simulink model "Controlador2"  (R2026a)
settings: Solver=VariableStepAuto  StopTime=tfin
values from neighbouring files (symbols this model uses):
  tesc = 5    [CodigoTurner.m]    (also in CodigoTurnerPerturbacion.m; FiguraModeloH.m; FiguraModeloMoro.m; FiguraModeloTurner.m)
libraries: slpidlib x1, realtime_pacer_lib x1
settings Model: Creator=Nehir RT  LastModifiedBy=Nehir RT

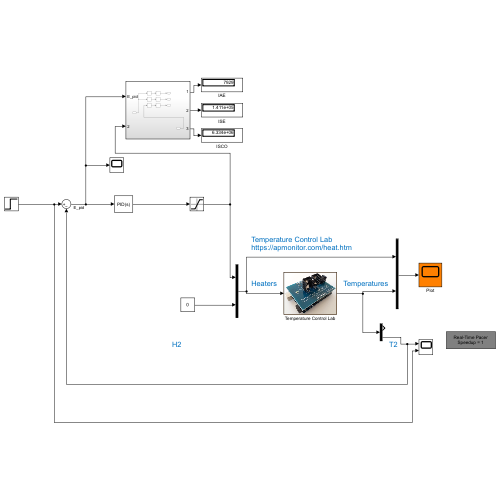
[thumbnail: Simulink's stored preview of the top-level diagram]
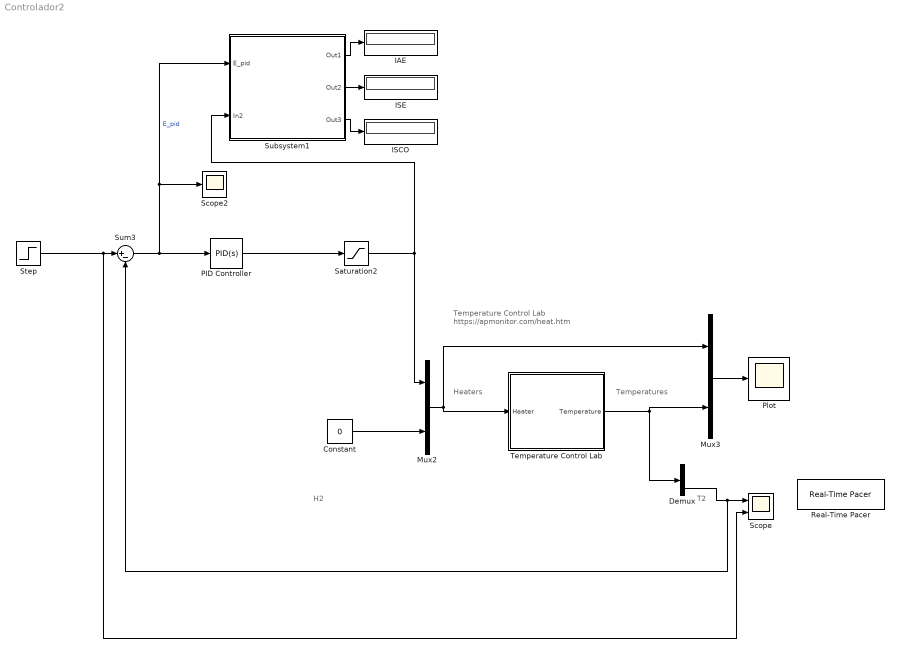
== system Controlador2 ==
  note: Temperatures
  note: Temperature Control Lab
      | https://apmonitor.com/heat.htm
  note: Heaters
  note: H2
  note: T2
  Constant : Constant  Value=0
  Demux : Demux  Outputs=2
  IAE : Display
  ISCO : Display
  ISE : Display
  Mux2 : Mux  Inputs=2
  Mux3 : Mux  Inputs=2
  PID Controller : slpidlib/PID Controller  Controller=PID  Form=Ideal  TimeDomain=Continuous-time  UseExternalTs=off  SampleTime=-1  IntegratorMethod=Forward Euler  FilterMethod=Forward Euler  ControllerParametersSource=internal  P=1.22923446994077  I=0.00854516737212471  UseKiTs=off  D=0  UseExternalDerivativeSource=off  N=100  UseFilter=on  TunerSelectOption=Transfer Function Based (PID Tuner App)  InitialConditionSource=internal  InitialConditionForIntegrator=0  InitialConditionForFilter=0  DifferentiatorICPrevScaledInput=0  ExternalReset=none  TrackingMode=off  Kt=1  LimitOutput=off  SatLimitsSource=internal  UpperSaturationLimit=inf  LowerSaturationLimit=-inf  LinearizeAsGain=on  AntiWindupMode=none  Kb=1  LimitIntegrator=off  UpperIntegratorSaturationLimit=inf  LowerIntegratorSaturationLimit=-inf  POutMin=[]  POutMax=[]  IOutMin=[]  IOutMax=[]  DOutMin=[]  DOutMax=[]  NOutMin=[]  NOutMax=[]  SumOutMin=[]  SumOutMax=[]  SaturationOutMin=[]  SaturationOutMax=[]  PParamMin=[]  PParamMax=[]  IParamMin=[]  IParamMax=[]  DParamMin=[]  DParamMax=[]  NParamMin=[]  NParamMax=[]  KbParamMin=[]  KbParamMax=[]  KtParamMin=[]  KtParamMax=[]  KbOutMin=[]  KbOutMax=[]  KtOutMin=[]  KtOutMax=[]  IntegratorOutMin=[]  IntegratorOutMax=[]  FilterOutMin=[]  FilterOutMax=[]  SumI1OutMin=[]  SumI1OutMax=[]  SumI2OutMin=[]  SumI2OutMax=[]  SumI3OutMin=[]  SumI3OutMax=[]  SumI4OutMin=[]  SumI4OutMax=[]  SumDOutMin=[]  SumDOutMax=[]  DifferentiatorOutMin=[]  DifferentiatorOutMax=[]  FilterDiffOutCoefMin=[]  FilterDiffOutCoefMax=[]  ReciprocalOutMin=[]  ReciprocalOutMax=[]  SumDenOutMin=[]  SumDenOutMax=[]  SumNumOutMin=[]  SumNumOutMax=[]  DivideOutMin=[]  DivideOutMax=[]  UdiffTsProdOutMin=[]  UdiffTsProdOutMax=[]  NTsProdOutMin=[]  NTsProdOutMax=[]  UintegralTsProdOutMin=[]  UintegralTsProdOutMax=[]  UngainTsProdOutMin=[]  UngainTsProdOutMax=[]  ClampingZeroOutDataTypeStr=Inherit: Inherit via back propagation  ClampingZeroOutMin=[]  ClampingZeroOutMax=[]  FilterDenConstantOutDataTypeStr=Inherit: Inherit via back propagation  FilterDenConstantOutMin=[]  FilterDenConstantOutMax=[]  PCopyOutDataTypeStr=Inherit: Inherit via back propagation  PCopyOutMin=[]  PCopyOutMax=[]  NCopyOutDataTypeStr=Inherit: Inherit via back propagation  NCopyOutMin=[]  NCopyOutMax=[]  IntegratorContinuousStateAttributes=''  IntegratorStateMustResolveToSignalObject=off  IntegratorRTWStateStorageClass=Auto  FilterContinuousStateAttributes=''  FilterStateMustResolveToSignalObject=off  FilterRTWStateStorageClass=Auto  ParallelPVariant=Passthrough  IdealPVariant=InternalParameters  IVariant=InternalParameters  DVariant=InternalParameters  IntegratorVariant=Continuous  SatVariant=Disabled  AWVariant=Passthrough  PCopyVariant=Disabled  TRVariant=Disabled  FdbkBlocksVariant=Forward  IdealPFdbkVariant=Disabled  SatFdbkVariant=Disabled  DerivativeFilterVariant=ContFilter  NVariant=InternalParameters  NCopyVariant=Disabled  FilterICVariant=InternalICsFilter  IntegratorICVariant=InternalICs  ExternalResetVariant=Disabled  TRSumVariant=Passthrough  SumFdbkVariant=Disabled  SumVariant=Sum_PID  TsampFilterVariant=InternalTs  TsampNgainVariant=Passthrough  TsampIntegralVariant=Disabled_SignalSpec  ExternalSaturationOutDataTypeStr=Inherit: Same as second input  DerivativeSourceVariant=ErrorSignal  PreIntVariant=InternalPreInt
  Plot : Scope
      settings: ActiveDisplayYMinimum=-12.499999999999996  ActiveDisplayYMaximum=112.5  DataLoggingSaveFormat=Array
  Real-Time Pacer : realtime_pacer_lib/Real-Time Pacer  simTimePerRealTime=1
      settings: SourceProductName=Real-Time Pacer
  Saturation2 : Saturate  UpperLimit=100  LowerLimit=0
  Scope : Scope  NumInputPorts=2
      settings: ActiveDisplayYMinimum=-6.8853861192570847  ActiveDisplayYMaximum=61.968475073313776  DataLoggingVariableName=DatosOut
  Scope2 : Scope
      settings: ActiveDisplayYMinimum=-4.9999999999999991  ActiveDisplayYMaximum=45  DataLoggingVariableName=ScopeData2
  Step : Step  Time=tesc  FinalValue=A  SampleTime=0
  Subsystem1 : Subsystem
  Sum3 : Sum  Inputs=|+-
  Temperature Control Lab : Subsystem
      mask Display: image('tclab.png');
  wires:
  PID Controller/1 -> Saturation2/1
  Saturation2/1 -> Mux2/1, Subsystem1/2(In2)
  Temperature Control Lab/1(Temperature) -> Mux3/2, Demux/1
  Demux/2 -> Sum3/2, Scope/1
  Mux2/1 -> Mux3/1, Temperature Control Lab/1(Heater)
  Step/1 -> Sum3/1, Scope/2
  Constant/1 -> Mux2/2
  Sum3/1 -> Scope2/1, Subsystem1/1(E_pid), PID Controller/1  "E_pid"
  Mux3/1 -> Plot/1
  Subsystem1/1(Out1) -> IAE/1
  Subsystem1/3(Out3) -> ISCO/1
  Subsystem1/2(Out2) -> ISE/1

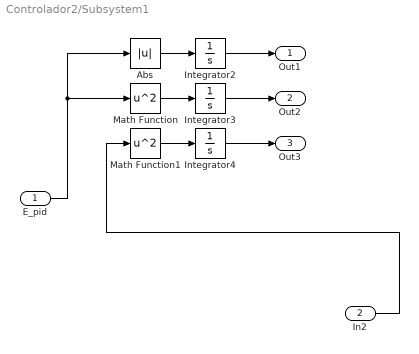
== system Controlador2/Subsystem1 ==
  E_pid : Inport
  In2 : Inport  Port=2
  Abs : Abs  SaturateOnIntegerOverflow=off
  Integrator2 : Integrator
  Integrator3 : Integrator
  Integrator4 : Integrator
  Math Function : Math  Operator=square
  Math Function1 : Math  Operator=square
  Out1 : Outport
  Out2 : Outport  Port=2
  Out3 : Outport  Port=3
  wires:
  E_pid/1 -> Math Function/1, Abs/1
  Math Function/1 -> Integrator3/1
  Integrator4/1 -> Out3/1
  Abs/1 -> Integrator2/1
  Math Function1/1 -> Integrator4/1
  Integrator3/1 -> Out2/1
  In2/1 -> Math Function1/1
  Integrator2/1 -> Out1/1

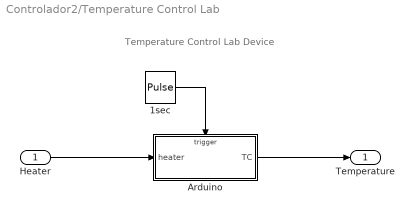
== system Controlador2/Temperature Control Lab ==
  note: Temperature Control Lab Device
  Heater : Inport
  1sec : DiscretePulseGenerator  PulseType=Time based  Period=1  PulseWidth=50
  Arduino : Subsystem  TreatAsAtomicUnit=on
  Temperature : Outport  VectorParamsAs1DForOutWhenUnconnected=off
  wires:
  1sec/1 -> Arduino/Trigger
  Arduino/1(TC) -> Temperature/1
  Heater/1 -> Arduino/1(heater)

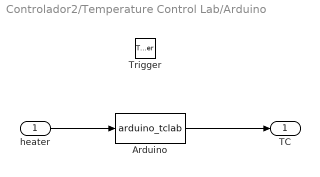
== system Controlador2/Temperature Control Lab/Arduino ==
  heater : Inport  LatchByDelayingOutsideSignal=on
  Trigger : TriggerPort  VariantControl=Variant
  Arduino : MATLABFcn  MATLABFcn=arduino_tclab
  TC : Outport  InitialOutput=[23 23]  VectorParamsAs1DForOutWhenUnconnected=off
  wires:
  heater/1 -> Arduino/1
  Arduino/1 -> TC/1
